simulink model "experiment101"  (R2018b)
settings: Solver=VariableStepAuto  StartTime=0.0  StopTime=10.0  RelTol=1e-3
settings Model: Creator=HIT-QJ  LastModifiedBy=HIT-QJ

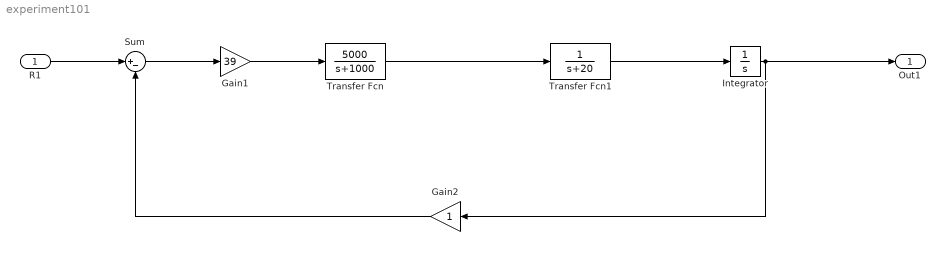
== system experiment101 ==
  R1 : Inport
  "Gain1 " : Gain  Gain=39
  "Gain2 " : Gain
  Integrator : Integrator
  Sum : Sum  Inputs=|+-
  Transfer Fcn : TransferFcn  Numerator=[5000]  Denominator=[1 1000]
  Transfer Fcn1 : TransferFcn  Denominator=[1 20]
  Out1 : Outport
  wires:
  R1/1 -> Sum/1
  Sum/1 -> "Gain1 "/1
  "Gain1 "/1 -> Transfer Fcn/1
  Transfer Fcn/1 -> Transfer Fcn1/1
  Transfer Fcn1/1 -> Integrator/1
  Integrator/1 -> "Gain2 "/1, Out1/1
  "Gain2 "/1 -> Sum/2
